simulink model "Forward_Kinematics"  (R2021b)
settings: Solver=VariableStepAuto  StartTime=0.0  StopTime=10.0  RelTol=1e-3
settings Model: Creator=Khaled  LastModifiedBy=Khaled

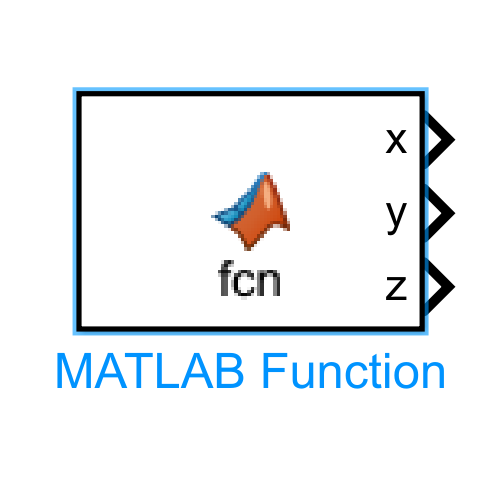
[thumbnail: Simulink's stored preview of the top-level diagram]
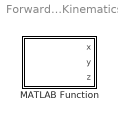
== system Forward_Kinematics ==
  MATLAB Function : MATLAB Function  TreatAsAtomicUnit=on

== matlab function Forward_Kinematics/MATLAB Function ==
  data: x output; y output; z output
function [x,y,z] = fcn()
B = forward_kinematics_func()
x = B(1,1);
y = B(2,1);
z = B(3,1);
end
